simulink model "lqgwork"  (R2020b)
settings: Solver=VariableStepAuto  StartTime=0.0  StopTime=100  RelTol=1e-3
undefined symbols (not defined in the file or in its folder): A15, B, Continuous, K, Time
libraries: ctrlSharedLib x1
settings Model: Creator=golam  LastModifiedBy=golam

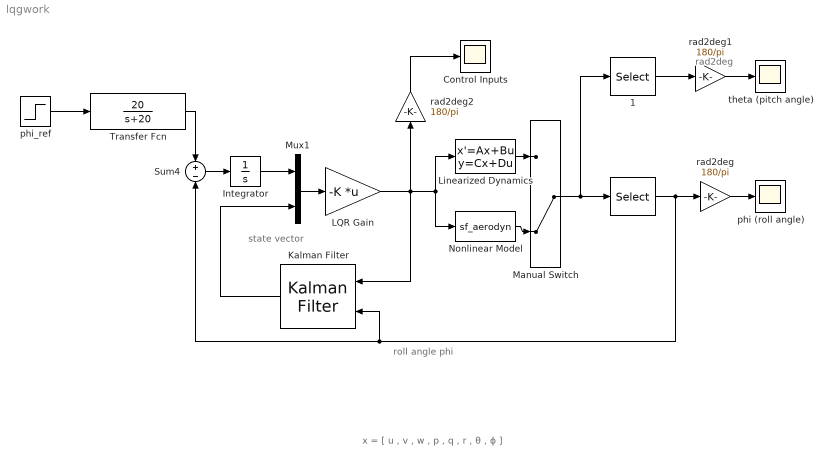
== system lqgwork ==
  note: x = [ u , v , w , p , q , r , θ , ϕ ]
  note: roll angle phi
  note: state vector
  note: rad2deg
  " " : Selector  InputPortWidth=8  IndexOptions=Index vector (dialog)  Indices=8  OutputSizes=1
  " 1" : Selector  InputPortWidth=8  IndexOptions=Index vector (dialog)  Indices=7  OutputSizes=1
  Control Inputs : Scope
  Integrator : Integrator
  Kalman Filter : ctrlSharedLib/Kalman Filter  TimeDomain=Continuous-Time  UseCurrentEstimator=on  ModelSource=Individual A, B, C, D matrices  ModelSourceVariable=ss(0.95,1,1,0,1)  A=A15  B=B  C=[0 0 0 0 0 0 0 1]  D=zeros(1,4)  NumberOfStates=8  NumberOfInputs=4  NumberOfOutputs=1  InitialEstimateSource=Dialog  X0=0  P0=10  UseK=off  UseGH=off  NumberOfProcessNoiseInputs=1  G=1  TimeInvariantG=on  H=0  TimeInvariantH=on  Q=0.001*eye(8)  TimeInvariantQ=on  R=0.001  TimeInvariantR=on  N=0  TimeInvariantN=on  AddInputPort=on  AddEnablePort=off  OutputEstimatedY=off  OutputP=off  Ts=-1
  LQR Gain : Gain  Gain=-K  Multiplication=Matrix(K*u)  SaturateOnIntegerOverflow=on  OutDataTypeStr=Inherit: Same as input  ParamDataTypeStr=Inherit: Same as input
  Linearized Dynamics : StateSpace  A=A15  B=B  C=eye(8)  D=zeros(8,4)  InitialCondition=0
  Manual Switch : ManualSwitch  CurrentSetting=0
  Mux1 : Mux  Inputs=2
  Nonlinear Model : S-Function  FunctionName=sf_aerodyn  SFunctionDeploymentMode=off  EnableBusSupport=off
  Sum4 : Sum  Inputs=+-  InputSameDT=on  SaturateOnIntegerOverflow=on  OutDataTypeStr=Inherit: Same as first input
  Transfer Fcn : TransferFcn  Numerator=20  Denominator=[1 20]
  phi (roll angle) : Scope
  phi_ref : Step  Time=0  After=pi/3  SampleTime=0
  rad2deg : Gain  Gain=180/pi  SaturateOnIntegerOverflow=on  OutDataTypeStr=Inherit: Same as input  ParamDataTypeStr=Inherit: Same as input
  rad2deg1 : Gain  Gain=180/pi  SaturateOnIntegerOverflow=on  OutDataTypeStr=Inherit: Same as input  ParamDataTypeStr=Inherit: Same as input
  rad2deg2 : Gain  Gain=180/pi  SaturateOnIntegerOverflow=on  OutDataTypeStr=Inherit: Same as input  ParamDataTypeStr=Inherit: Same as input
  theta (pitch angle) : Scope
  wires:
  phi_ref/1 -> Transfer Fcn/1
  Transfer Fcn/1 -> Sum4/1
  Linearized Dynamics/1 -> Manual Switch/1
  Sum4/1 -> Integrator/1
  LQR Gain/1 -> Kalman Filter/1, Linearized Dynamics/1, Nonlinear Model/1, rad2deg2/1
  rad2deg2/1 -> Control Inputs/1
  rad2deg1/1 -> theta (pitch angle)/1
  rad2deg/1 -> phi (roll angle)/1
  " 1"/1 -> rad2deg1/1
  Nonlinear Model/1 -> Manual Switch/2
  Mux1/1 -> LQR Gain/1
  Integrator/1 -> Mux1/1
  " "/1 -> rad2deg/1, Sum4/2, Kalman Filter/2
  Manual Switch/1 -> " "/1, " 1"/1
  Kalman Filter/1 -> Mux1/2
